simulink subsystem "PvtSubSys_VSM_LCKIE"  (R2020b)
settings: Solver=VariableStepAuto  StartTime=0.0  StopTime=10.0  RelTol=1e-3
values from neighbouring files (symbols this model uses):
  P_VSM_LCKIE_ClassInput = 0.0    [LCKIE.sldd]
  P_VSM_LCKIE_Laneoffset : value not decoded    [LCKIE.sldd]
  P_VSM_LCKIE_Laneoffset_BP : value not decoded    [LCKIE.sldd]
  P_VSM_LCKIE_LatC_DisOffofLanWidth : value not decoded    [LCKIE.sldd]
  P_VSM_LCKIE_LatC_DisOffofSpd : value not decoded    [LCKIE.sldd]
  P_VSM_LCKIE_LatC_DisSW = 0.0    [LCKIE.sldd]
  P_VSM_LCKIE_LatC_LanWidth : value not decoded    [LCKIE.sldd]
  P_VSM_LCKIE_LATC_LimitDis : value not decoded    [LCKIE.sldd]
  P_VSM_LCKIE_LATC_LimitDis_BP : value not decoded    [LCKIE.sldd]
  P_VSM_LCKIE_LatC_LimitDisEgoToObjSelt = 1.5    [LCKIE.sldd]
  P_VSM_LCKIE_LatC_LimitEgoToOppLane = 0.3    [LCKIE.sldd]
  P_VSM_LCKIE_LatC_maxLimitDisREToLane = 2.5    [LCKIE.sldd]
  P_VSM_LCKIE_LatC_minLimitDisREToLane = 1.2    [LCKIE.sldd]
  P_VSM_LCKIE_LatC_MoveEnableDis = 0.0    [LCKIE.sldd]
  P_VSM_LCKIE_LatC_RESafDis = 0.8    [LCKIE.sldd]
  P_VSM_LCKIE_LatC_SafeDisofLanWidth : value not decoded    [LCKIE.sldd]
  P_VSM_LCKIE_LatC_Spd : value not decoded    [LCKIE.sldd]
  P_VSM_LCKIE_LongC_d1 : value not decoded    [LCKIE.sldd]
  P_VSM_LCKIE_LongC_d2 : value not decoded    [LCKIE.sldd]
  P_VSM_LCKIE_LongC_DetaSpd : value not decoded    [LCKIE.sldd]
  P_VSM_LCKIE_LongC_DirecChangeDis = 20.0    [LCKIE.sldd]
  P_VSM_LCKIE_LongC_FleetOff = 80.0    [LCKIE.sldd]
  P_VSM_LCKIE_LongC_maxDis = 80.0    [LCKIE.sldd]
  P_VSM_LCKIE_LongC_minDis = 50.0    [LCKIE.sldd]
  P_VSM_LCKIE_LongC_ShutDownLongDis = -25.0    [LCKIE.sldd]
  P_VSM_LCKIE_LongC_ShutDownTTC = -4.0    [LCKIE.sldd]
  P_VSM_LCKIE_LongC_Spd : value not decoded    [LCKIE.sldd]
  P_VSM_LCKIE_LongC_toff = 10.0    [LCKIE.sldd]
  P_VSM_LCKIE_OFC_ActDis = 10.0    [LCKIE.sldd]
  P_VSM_LCKIE_OFC_DownDis = 10.0    [LCKIE.sldd]
  P_VSM_LCKIE_OFC_DownTTC = 5.0    [LCKIE.sldd]
  P_VSM_LCKIE_OFC_SafDis = 10.0    [LCKIE.sldd]
  P_VSM_LCKIE_OFC_Toff = 3.0    [LCKIE.sldd]
  P_VSM_LCKIE_ORC_LatDis = 1.8    [LCKIE.sldd]
  P_VSM_LCKIE_ORC_LimitDis1 = -30.0    [LCKIE.sldd]
  P_VSM_LCKIE_ORC_LimitDis2 = -10.0    [LCKIE.sldd]
  P_VSM_LCKIE_ORC_LimitTTC = 10.0    [LCKIE.sldd]
  P_VSM_LCKIE_ORC_LowSpd = -5.0    [LCKIE.sldd]
  P_VSM_LCKIE_POC_Delaytime : value not decoded    [LCKIE.sldd]
  P_VSM_LCKIE_POC_detaSpd : value not decoded    [LCKIE.sldd]
  P_VSM_LCKIE_POC_LimitDis = -15.0    [LCKIE.sldd]
  P_VSM_LCKIE_POC_LimitTTC = 2.0    [LCKIE.sldd]
  P_VSM_LCKIE_State_CurveMax = 0.005    [LCKIE.sldd]
  P_VSM_LCKIE_State_CurveMin = 0.0055555555555555558    [LCKIE.sldd]
  P_VSM_LCKIE_State_detaspd = 1.39    [LCKIE.sldd]
  P_VSM_LCKIE_State_detaspd_enable = 1.0    [LCKIE.sldd]
  P_VSM_LCKIE_State_DriverInputTrqValue_enable = 1.0    [LCKIE.sldd]
  P_VSM_LCKIE_State_ELKObjClc = 1.0    [LCKIE.sldd]
  P_VSM_LCKIE_State_HWASts_disable = 1.0    [LCKIE.sldd]
  P_VSM_LCKIE_State_IEObjClc = 1.0    [LCKIE.sldd]
  P_VSM_LCKIE_State_IFVReady = 1.0    [LCKIE.sldd]
  P_VSM_LCKIE_State_lamb_enable = 1.0    [LCKIE.sldd]
  P_VSM_LCKIE_State_Lanecurve_enable = 1.0    [LCKIE.sldd]
  P_VSM_LCKIE_State_LaneWidth_enable = 1.0    [LCKIE.sldd]
  P_VSM_LCKIE_State_Off2on = 3.0    [LCKIE.sldd]
  P_VSM_LCKIE_State_OppObjClc = 1.0    [LCKIE.sldd]
  P_VSM_LCKIE_STATE_ORCObjenable = 0.0    [LCKIE.sldd]
  P_VSM_LCKIE_State_Vehspeed_enable = 1.0    [LCKIE.sldd]
  P_VSM_LCKIE_State_wiper_enable = 1.0    [LCKIE.sldd]
  P_VSM_LCKIE_tcycle = 0.02    [LCKIE.sldd]
undefined symbols (not defined in the file or in its folder): P_Global_Vehicle_Length_m, P_Global_VehicleWidthMin_m, P_VSM_LSMC_SampleTime, STATE
libraries: simulink x62
(part 3 of 5)

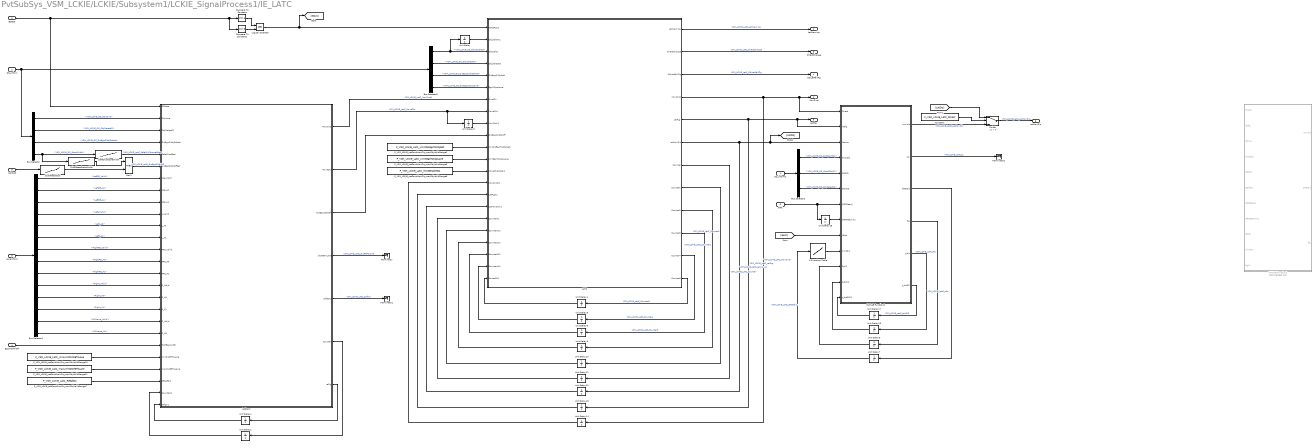
== system PvtSubSys_VSM_LCKIE/LCKIE/Subsystem1/LCKIE_SignalProcess1/IE_LATC ==
  OS_Inform : Inport
  IEstate : Inport  Port=2
  VehSpd : Inport  Port=3
  EgoHalfWidth : Inport  Port=4
  LaneInform : Inport  Port=5
  ORC : Inport  Port=6
  1-D Lookup Table : Lookup_n-D  NumberOfTableDimensions=1  BreakpointsForDimension1=P_VSM_LCKIE_LATC_LimitDis_BP  Table=P_VSM_LCKIE_LATC_LimitDis  InternalRulePriority=Speed  RndMeth=Simplest  InputSameDT=on
  Bus Selector : BusSelector  OutputSignals=VSM_LCKIE_OS_ObjLane,VSM_LCKIE_OS_ObjSelectID,VSM_LCKIE_OS_DisEgo2ObjSelect,VSM_LCKIE_OS_RoadWidth
  Bus Selector1 : BusSelector  OutputSignals=Lanes.LeftRE_Valid,Lanes.LeftRE_A0,Lanes.LeftRE_A1,Lanes.Left_Valid,Lanes.Left_A0,Lanes.Left_A1,Lanes.RightRE_Valid,Lanes.RightRE_A0,Lanes.RightRE_A1,Lanes.Right_Valid,Lanes.Right_A0,Lanes.Right_A1,Center.LCKLane_Valid,Center.LCKLane_A0
  Bus Selector2 : BusSelector  OutputSignals=VSM_LCKIE_OS_DisEgo2Obj,VSM_LCKIE_OS_OppRObjID,VSM_LCKIE_OS_ObjSelectID
  Bus Selector3 : BusSelector  OutputSignals=VSM_LCKIE_OS_ObjIDSelect,VSM_LCKIE_OS_ObjSelectID,VSM_LCKIE_OS_DisEgo2ObjSelect,VSM_LCKIE_OS_DisEgo2OppLane
  Compare To Constant : simulink/Logic and Bit Operations/Compare To Constant  relop===  const=4  OutDataTypeStr=boolean
  Compare To Constant1 : simulink/Logic and Bit Operations/Compare To Constant  relop===  const=5  OutDataTypeStr=boolean
  Constant : Constant  Value=P_VSM_LCKIE_LatC_DisSW
  DisOffsetofLaneWidth : Lookup_n-D  NumberOfTableDimensions=1  BreakpointsForDimension1=P_VSM_LCKIE_LatC_LanWidth  Table=P_VSM_LCKIE_LatC_DisOffofLanWidth  ExtrapMethod=Clip  UseLastTableValue=on  InternalRulePriority=Speed  RndMeth=Simplest  InputSameDT=on
  DisOffsetofSpd : Lookup_n-D  NumberOfTableDimensions=1  BreakpointsForDimension1=P_VSM_LCKIE_LatC_Spd  Table=P_VSM_LCKIE_LatC_DisOffofSpd  ExtrapMethod=Clip  UseLastTableValue=on  InternalRulePriority=Speed  RndMeth=Simplest  InputSameDT=on
  LATC : MATLAB Function  TreatAsAtomicUnit=on
  LatParm : MATLAB Function  TreatAsAtomicUnit=on
  Logical Operator : Logic  Operator=OR  AllPortsSameDT=off  OutDataTypeStr=boolean
  MATLAB Function1 : MATLAB Function  Commented=on  TreatAsAtomicUnit=on
  MATLAB Function2 : MATLAB Function  TreatAsAtomicUnit=on
  Max1 : MinMax  Function=max  Inputs=2
  OS_Inform1 : InportShadow
  P_VSM_LCKIE_LatConditionClc_maxObjValidRange10 : Constant  Value=P_VSM_LCKIE_LatC_minLimitDisREToLane
  P_VSM_LCKIE_LatConditionClc_maxObjValidRange11 : Constant  Value=P_VSM_LCKIE_LatC_maxLimitDisREToLane
  P_VSM_LCKIE_LatConditionClc_maxObjValidRange2 : Constant  Value=P_VSM_LCKIE_LatC_LimitDisEgoToObjSelt
  P_VSM_LCKIE_LatConditionClc_maxObjValidRange3 : Constant  Value=P_VSM_LCKIE_LatC_LimitEgoToOppLane
  P_VSM_LCKIE_LatConditionClc_maxObjValidRange7 : Constant  Value=P_VSM_LCKIE_LatC_RESafDis
  P_VSM_LCKIE_LatConditionClc_maxObjValidRange8 : Constant  Value=P_VSM_LCKIE_LatC_MoveEnableDis  OutDataTypeStr=single
  SafeDisofLaneWidth : Lookup_n-D  NumberOfTableDimensions=1  BreakpointsForDimension1=P_VSM_LCKIE_LatC_LanWidth  Table=P_VSM_LCKIE_LatC_SafeDisofLanWidth  ExtrapMethod=Clip  UseLastTableValue=on  InternalRulePriority=Speed  RndMeth=Simplest  InputSameDT=on
  Switch : Switch  Criteria=u2 > Threshold
  Terminator : Terminator
  Terminator1 : Terminator
  Terminator2 : Terminator
  Unit Delay{,1..17} (18 alike) : UnitDelay  SampleTime=-1  HasFrameUpgradeWarning=on
  MovDirct : Outport
  LatWarning : Outport  Port=2
  DirectChange : Outport  Port=3
  ObjLatFailFlg : Outport  Port=4
  LatFLg : Outport  Port=5
  LatMovDis : Outport  Port=6
  wires:
  DisOffsetofLaneWidth/1 -> Max1/1
  IEstate/1 -> LatParm/1(IEState), Compare To Constant1/1, Compare To Constant/1
  EgoHalfWidth/1 -> LatParm/21(HalfEgoWidth)
  Max1/1 -> LatParm/6(DisEgo2ObjOffset)  "VSM_LCKIE_LatC_DisEgo2ObjOff"
  SafeDisofLaneWidth/1 -> LatParm/5(SafeDisoffset)  "VSM_LCKIE_LatC_SafeDisToLaneEdge"
  Bus Selector/4 -> SafeDisofLaneWidth/1, DisOffsetofLaneWidth/1  "<VSM_LCKIE_OS_RoadWidth>"
  DisOffsetofSpd/1 -> Max1/2
  VehSpd/1 -> DisOffsetofSpd/1
  OS_Inform/1 -> Bus Selector3/1, Bus Selector/1
  Bus Selector/1 -> LatParm/2(ObjLane)  "<VSM_LCKIE_OS_ObjLane>"
  Bus Selector/2 -> LatParm/3(ObjSelectID)  "<VSM_LCKIE_OS_ObjSelectID>"
  LaneInform/1 -> Bus Selector1/1
  Bus Selector1/2 -> LatParm/8(LRe_A0)  "<LeftRE_A0>"
  Bus Selector1/3 -> LatParm/9(LRe_A1)  "<LeftRE_A1>"
  Bus Selector1/1 -> LatParm/7(LRe_Valid)  "<LeftRE_Valid>"
  Bus Selector1/4 -> LatParm/10(L_Valid)  "<Left_Valid>"
  Bus Selector1/5 -> LatParm/11(L_A0)  "<Left_A0>"
  Bus Selector1/6 -> LatParm/12(L_A1)  "<Left_A1>"
  Bus Selector1/7 -> LatParm/13(RRe_Valid)  "<RightRE_Valid>"
  Bus Selector1/8 -> LatParm/14(RRe_A0)  "<RightRE_A0>"
  Bus Selector1/9 -> LatParm/15(RRe_A1)  "<RightRE_A1>"
  Bus Selector1/10 -> LatParm/16(R_Valid)  "<Right_Valid>"
  Bus Selector1/11 -> LatParm/17(R_A0)  "<Right_A0>"
  Bus Selector1/12 -> LatParm/18(R_A1)  "<Right_A1>"
  Bus Selector1/13 -> LatParm/19(C_Valid)  "<LCKLane_Valid>"
  Bus Selector1/14 -> LatParm/20(C_A0)  "<LCKLane_A0>"
  P_VSM_LCKIE_LatConditionClc_maxObjValidRange10/1 -> LatParm/22(minDisREToLane)
  P_VSM_LCKIE_LatConditionClc_maxObjValidRange11/1 -> LatParm/23(maxDisREToLane)
  LatParm/7(reflg) -> Unit Delay1/1
  Unit Delay1/1 -> LatParm/26(reflgK1)
  Unit Delay2/1 -> LatParm/25(CounterK1)
  LatParm/6(Counter) -> Unit Delay2/1
  Bus Selector/3 -> LatParm/4(DisEgo2ObjSelect)  "<VSM_LCKIE_OS_DisEgo2ObjSelect>"
  P_VSM_LCKIE_LatConditionClc_maxObjValidRange7/1 -> LatParm/24(RESafDis)
  Bus Selector3/1 -> Unit Delay/1, LATC/3(ObjSelID)  "<VSM_LCKIE_OS_ObjIDSelect>"
  Bus Selector3/2 -> LATC/4(ObjSelectID)  "<VSM_LCKIE_OS_ObjSelectID>"
  Bus Selector3/3 -> LATC/5(DisEgo2ObjSelt)  "<VSM_LCKIE_OS_DisEgo2ObjSelect>"
  Bus Selector3/4 -> LATC/6(Ego2OppLane)  "<VSM_LCKIE_OS_DisEgo2OppLane>"
  Unit Delay/1 -> LATC/2(ObjSelIDK1)
  LatParm/1(MovDirct) -> LATC/7(DirctClc)  "VSM_LCKIE_LatC_MovDirct1"
  LatParm/2(MoveDis) -> Unit Delay3/1, LATC/8(MoveDis)  "VSM_LCKIE_LatC_MoveDis"
  LatParm/3(DisEgo2ObjOff) -> LATC/10(DisEgo2oObjOff)
  P_VSM_LCKIE_LatConditionClc_maxObjValidRange2/1 -> LATC/11(minDisEgoToObjSelt)
  P_VSM_LCKIE_LatConditionClc_maxObjValidRange3/1 -> LATC/12(minEgoToOppLane)
  P_VSM_LCKIE_LatConditionClc_maxObjValidRange8/1 -> LATC/13(MoveEnableDis)
  Unit Delay3/1 -> LATC/9(MovDisK1)
  LATC/12(Counter5) -> Unit Delay4/1  "VSM_LCKIE_LatC_Counter5"
  Unit Delay4/1 -> LATC/22(Couter5K1)
  LATC/11(Counter4) -> Unit Delay5/1  "VSM_LCKIE_LatC_Counter4"
  Unit Delay5/1 -> LATC/21(Counter4K1)
  LATC/10(Counter3) -> Unit Delay8/1  "VSM_LCKIE_LatC_Counter3"
  Unit Delay8/1 -> LATC/20(Counter3K1)
  LATC/9(Counter2) -> Unit Delay9/1  "VSM_LCKIE_LatC_Counter2"
  Unit Delay9/1 -> LATC/19(Counter2K1)
  LATC/8(Counter1) -> Unit Delay10/1  "VSM_LCKIE_LatC_Counter1"
  Unit Delay10/1 -> LATC/18(Counter1K1)
  LATC/7(Counter) -> Unit Delay11/1  "VSM_LCKIE_LatC_Counter"
  Unit Delay11/1 -> LATC/17(CounterK1)
  LATC/6(LatMovDis) -> Unit Delay12/1, MATLAB Function2/3(latmov), [LatDis]  "VSM_LCKIE_LatC_latmovori"
  Unit Delay12/1 -> LATC/16(LatMovDisK1)
  LATC/5(LatFLg) -> MATLAB Function2/2(latflg), LatFLg/1, Unit Delay13/1  "VSM_LCKIE_LatC_LatFLg"
  Unit Delay13/1 -> LATC/15(LatFLgK1)
  LATC/4(MovDirct) -> MATLAB Function2/1(Direct), MovDirct/1, Unit Delay14/1  "VSM_LCKIE_LatC_MovDirct"
  Unit Delay14/1 -> LATC/14(MovDirctK1)
  LatParm/4(DisREToLane) -> Terminator/1  "VSM_LCKIE_LatC_DisREToLane"
  LatParm/5(SafeDis) -> Terminator1/1  "VSM_LCKIE_LatC_SafDis"
  LATC/1(LatWarning) -> LatWarning/1  "VSM_LCKIE_LatC_LatWarning"
  LATC/2(DirectChange) -> DirectChange/1  "VSM_LCKIE_LatC_DirectChange"
  LATC/3(ObjLatFailFlg) -> ObjLatFailFlg/1  "VSM_LCKIE_LatC_ObjLatFailFlg"
  Compare To Constant/1 -> Logical Operator/1
  Compare To Constant1/1 -> Logical Operator/2
  Logical Operator/1 -> [IEAct], LATC/1(IEActFlgK1)
  MATLAB Function2/1(movdis) -> Switch/3  "VSM_LCKIE_LatC_LatMovDis"
  OS_Inform1/1 -> Bus Selector2/1
  Bus Selector2/2 -> MATLAB Function2/5(ORCID)  "<VSM_LCKIE_OS_OppRObjID>"
  Bus Selector2/1 -> MATLAB Function2/4(Dis2Obj)  "<VSM_LCKIE_OS_DisEgo2Obj>"
  Bus Selector2/3 -> MATLAB Function2/6(SelctID)  "<VSM_LCKIE_OS_ObjSelectID>"
  ORC/1 -> MATLAB Function2/7(ORCReady), Unit Delay15/1
  1-D Lookup Table/1 -> MATLAB Function2/10(limitDis)
  MATLAB Function2/4(flg) -> Unit Delay6/1  "VSM_LCKIE_LatC_Flg"
  Unit Delay6/1 -> MATLAB Function2/11(flgK1)
  MATLAB Function2/3(detaDis) -> Unit Delay7/1
  Unit Delay7/1 -> 1-D Lookup Table/1  "VSM_LCKIE_LatC_DetaDis"
  Unit Delay15/1 -> MATLAB Function2/8(ORCReadyK1)
  [IEAct] -> MATLAB Function2/9(IEAct)
  Constant/1 -> Switch/2
  Switch/1 -> LatMovDis/1  "VSM_LCKIE_LatC_LatMovDis"
  [LatDis] -> Switch/1
  MATLAB Function2/6(t_disOR) -> Unit Delay17/1  "VSM_LCKIE_LatC_tdisOR"
  Unit Delay17/1 -> MATLAB Function2/13(t_disORK1)
  MATLAB Function2/5(t_dis) -> Unit Delay16/1  "VSM_LCKIE_LatC_tdis"
  Unit Delay16/1 -> MATLAB Function2/12(t_disK1)
  MATLAB Function2/2(t_s) -> Terminator2/1  "VSM_LCKIE_LatC_ts"

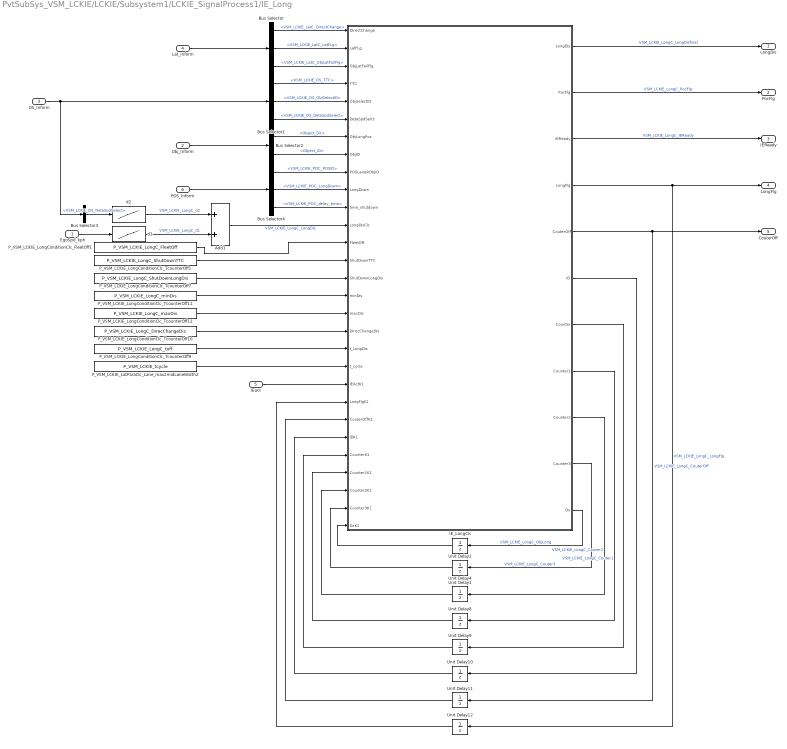
== system PvtSubSys_VSM_LCKIE/LCKIE/Subsystem1/LCKIE_SignalProcess1/IE_Long ==
  EgoSpd_kph : Inport
  Obj_Inform : Inport  Port=2
  OS_Inform : Inport  Port=3
  Lat_Inform : Inport  Port=4
  IEact : Inport  Port=5
  POS_Inform : Inport  Port=6
  Add1 : Sum
  Bus Selector : BusSelector  OutputSignals=VSM_LCKIE_LatC_DirectChange,VSM_LCKIE_LatC_LatFLg,VSM_LCKIE_LatC_ObjLatFailFlg
  Bus Selector1 : BusSelector  OutputSignals=VSM_LCKIE_OS_TTC,VSM_LCKIE_OS_ObjSelectID,VSM_LCKIE_OS_DetaSpdSelect
  Bus Selector2 : BusSelector  OutputSignals=Object_DX,Object_ID
  Bus Selector3 : BusSelector  OutputSignals=VSM_LCKIE_OS_DetaSpdSelect
  Bus Selector4 : BusSelector  OutputSignals=VSM_LCKIE_POC_POSID,VSM_LCKIE_POC_LongDown,VSM_LCKIE_POC_delay_time
  IE_LongClc : MATLAB Function  TreatAsAtomicUnit=on
  P_VSM_LCKIE_LatParaClc_Lane_max2midLaneWidth2 : Constant  Value=P_VSM_LCKIE_tcycle
  P_VSM_LCKIE_LongConditionClc_FleetOff1 : Constant  Value=P_VSM_LCKIE_LongC_FleetOff
  P_VSM_LCKIE_LongConditionClc_TcounterOff1 : Constant  Value=P_VSM_LCKIE_LongC_ShutDownTTC
  P_VSM_LCKIE_LongConditionClc_TcounterOff10 : Constant  Value=P_VSM_LCKIE_LongC_DirecChangeDis
  P_VSM_LCKIE_LongConditionClc_TcounterOff11 : Constant  Value=P_VSM_LCKIE_LongC_minDis
  P_VSM_LCKIE_LongConditionClc_TcounterOff12 : Constant  Value=P_VSM_LCKIE_LongC_maxDis
  P_VSM_LCKIE_LongConditionClc_TcounterOff7 : Constant  Value=P_VSM_LCKIE_LongC_ShutDownLongDis
  P_VSM_LCKIE_LongConditionClc_TcounterOff9 : Constant  Value=P_VSM_LCKIE_LongC_toff
  Unit Delay{1..2,4,8..12} (8 alike) : UnitDelay  SampleTime=-1  HasFrameUpgradeWarning=on
  d1 : Lookup_n-D  NumberOfTableDimensions=1  BreakpointsForDimension1=P_VSM_LCKIE_LongC_Spd  Table=P_VSM_LCKIE_LongC_d1  ExtrapMethod=Clip  UseLastTableValue=on  InternalRulePriority=Speed  RndMeth=Simplest  InputSameDT=on
  d2 : Lookup_n-D  NumberOfTableDimensions=1  BreakpointsForDimension1=P_VSM_LCKIE_LongC_DetaSpd  Table=P_VSM_LCKIE_LongC_d2  ExtrapMethod=Clip  UseLastTableValue=on  InternalRulePriority=Speed  OutDataTypeStr=single  RndMeth=Simplest  InputSameDT=on
  LongDis : Outport
  PocFlg : Outport  Port=2
  IEReady : Outport  Port=3
  LongFlg : Outport  Port=4
  CouterOff : Outport  Port=5
  wires:
  Bus Selector3/1 -> d2/1  "<VSM_LCKIE_OS_DetaSpdSelect>"
  EgoSpd_kph/1 -> d1/1
  d2/1 -> Add1/1  "VSM_LCKIE_LongC_d2"
  d1/1 -> Add1/2  "VSM_LCKIE_LongC_d1"
  Add1/1 -> IE_LongClc/12(LongDisClc)  "VSM_LCKIE_LongC_LongDis"
  Lat_Inform/1 -> Bus Selector/1
  OS_Inform/1 -> Bus Selector1/1, Bus Selector3/1
  P_VSM_LCKIE_LongConditionClc_TcounterOff1/1 -> IE_LongClc/14(ShutDownTTC)
  P_VSM_LCKIE_LongConditionClc_TcounterOff7/1 -> IE_LongClc/15(ShutDownLongDis)
  P_VSM_LCKIE_LongConditionClc_TcounterOff9/1 -> IE_LongClc/19(t_LongDis)
  P_VSM_LCKIE_LatParaClc_Lane_max2midLaneWidth2/1 -> IE_LongClc/20(t_cycle)
  IE_LongClc/10(Counter3) -> Unit Delay4/1  "VSM_LCKIE_LongC_Couter3"
  Unit Delay4/1 -> IE_LongClc/28(Counter3K1)
  IE_LongClc/9(Counter2) -> Unit Delay1/1  "VSM_LCKIE_LongC_Couter2"
  Unit Delay1/1 -> IE_LongClc/27(Counter2K1)
  IE_LongClc/8(Counter1) -> Unit Delay8/1  "VSM_LCKIE_LongC_Couter1"
  Unit Delay8/1 -> IE_LongClc/26(Counter1K1)
  IE_LongClc/7(Counter) -> Unit Delay9/1
  Unit Delay9/1 -> IE_LongClc/25(CounterK1)
  IE_LongClc/6(ID) -> Unit Delay10/1
  Unit Delay10/1 -> IE_LongClc/24(IDK1)
  IE_LongClc/5(CouterOff) -> CouterOff/1, Unit Delay11/1  "VSM_LCKIE_LongC_CouterOff"
  Unit Delay11/1 -> IE_LongClc/23(CouterOffK1)
  IE_LongClc/4(LongFlg) -> LongFlg/1, Unit Delay12/1  "VSM_LCKIE_LongC_LongFlg"
  Unit Delay12/1 -> IE_LongClc/22(LongFlgK1)
  IE_LongClc/3(IEReady) -> IEReady/1  "VSM_LCKIE_LongC_IEReady"
  Bus Selector/2 -> IE_LongClc/2(LatFLg)  "<VSM_LCKIE_LatC_LatFLg>"
  Bus Selector/3 -> IE_LongClc/3(ObjLatFailFlg)  "<VSM_LCKIE_LatC_ObjLatFailFlg>"
  Bus Selector1/2 -> IE_LongClc/5(ObjSelectID)  "<VSM_LCKIE_OS_ObjSelectID>"
  Bus Selector1/3 -> IE_LongClc/6(DetaSpdSelct)  "<VSM_LCKIE_OS_DetaSpdSelect>"
  Bus Selector1/1 -> IE_LongClc/4(TTC)  "<VSM_LCKIE_OS_TTC>"
  Obj_Inform/1 -> Bus Selector2/1
  Bus Selector2/2 -> IE_LongClc/8(ObjID)  "<Object_ID>"
  Bus Selector2/1 -> IE_LongClc/7(ObjLongPos)  "<Object_DX>"
  POS_Inform/1 -> Bus Selector4/1
  IE_LongClc/1(LongDis) -> LongDis/1  "VSM_LCKIE_LongC_LongDisfinal"
  IE_LongClc/2(PocFlg) -> PocFlg/1  "VSM_LCKIE_LongC_PocFlg"
  IE_LongClc/11(Dx) -> Unit Delay2/1  "VSM_LCKIE_LongC_ObjLong"
  P_VSM_LCKIE_LongConditionClc_FleetOff1/1 -> IE_LongClc/13(FleetOff)
  Unit Delay2/1 -> IE_LongClc/29(DxK1)
  P_VSM_LCKIE_LongConditionClc_TcounterOff11/1 -> IE_LongClc/16(minDis)
  P_VSM_LCKIE_LongConditionClc_TcounterOff12/1 -> IE_LongClc/17(maxDis)
  P_VSM_LCKIE_LongConditionClc_TcounterOff10/1 -> IE_LongClc/18(DirecChangeDis)
  Bus Selector4/1 -> IE_LongClc/9(POSLaneRObjID)  "<VSM_LCKIE_POC_POSID>"
  Bus Selector4/2 -> IE_LongClc/10(LongDown)  "<VSM_LCKIE_POC_LongDown>"
  Bus Selector4/3 -> IE_LongClc/11(time_shutdown)  "<VSM_LCKIE_POC_delay_time>"
  Bus Selector/1 -> IE_LongClc/1(DirectChange)  "<VSM_LCKIE_LatC_DirectChange>"
  IEact/1 -> IE_LongClc/21(IEActK1)

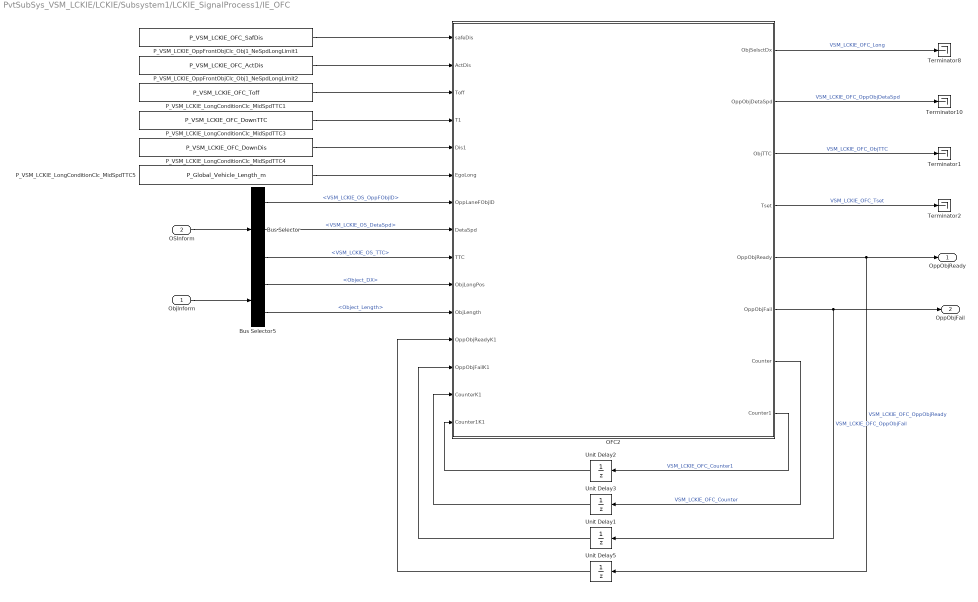
== system PvtSubSys_VSM_LCKIE/LCKIE/Subsystem1/LCKIE_SignalProcess1/IE_OFC ==
  ObjInform : Inport
  OSInform : Inport  Port=2
  Bus Selector : BusSelector  OutputSignals=VSM_LCKIE_OS_OppFObjID,VSM_LCKIE_OS_DetaSpd,VSM_LCKIE_OS_TTC
  Bus Selector5 : BusSelector  OutputSignals=Object_DX,Object_Length
  OFC2 : MATLAB Function  TreatAsAtomicUnit=on
  P_VSM_LCKIE_LongConditionClc_MidSpdTTC1 : Constant  Value=P_VSM_LCKIE_OFC_Toff
  P_VSM_LCKIE_LongConditionClc_MidSpdTTC3 : Constant  Value=P_VSM_LCKIE_OFC_DownTTC
  P_VSM_LCKIE_LongConditionClc_MidSpdTTC4 : Constant  Value=P_VSM_LCKIE_OFC_DownDis
  P_VSM_LCKIE_LongConditionClc_MidSpdTTC5 : Constant  Value=P_Global_Vehicle_Length_m
  P_VSM_LCKIE_OppFrontObjClc_Obj1_NeSpdLongLimit1 : Constant  Value=P_VSM_LCKIE_OFC_SafDis
  P_VSM_LCKIE_OppFrontObjClc_Obj1_NeSpdLongLimit2 : Constant  Value=P_VSM_LCKIE_OFC_ActDis
  Terminator{1..2,8,10} (4 alike) : Terminator
  Unit Delay{1..3,5} (4 alike) : UnitDelay  SampleTime=-1  HasFrameUpgradeWarning=on
  OppObjReady : Outport
  OppObjFail : Outport  Port=2
  wires:
  OFC2/3(ObjTTC) -> Terminator1/1  "VSM_LCKIE_OFC_ObjTTC"
  Unit Delay2/1 -> OFC2/15(Counter1K1)
  OFC2/8(Counter1) -> Unit Delay2/1  "VSM_LCKIE_OFC_Counter1"
  Bus Selector/3 -> OFC2/9(TTC)  "<VSM_LCKIE_OS_TTC>"
  Bus Selector/2 -> OFC2/8(DetaSpd)  "<VSM_LCKIE_OS_DetaSpd>"
  Bus Selector/1 -> OFC2/7(OppLaneFObjID)  "<VSM_LCKIE_OS_OppFObjID>"
  OSInform/1 -> Bus Selector/1
  Unit Delay5/1 -> OFC2/12(OppObjReadyK1)
  Unit Delay1/1 -> OFC2/13(OppObjFailK1)
  OFC2/2(OppObjDetaSpd) -> Terminator10/1  "VSM_LCKIE_OFC_OppObjDetaSpd"
  OFC2/6(OppObjFail) -> Unit Delay1/1, OppObjFail/1  "VSM_LCKIE_OFC_OppObjFail"
  OFC2/4(Tset) -> Terminator2/1  "VSM_LCKIE_OFC_Tset"
  Bus Selector5/1 -> OFC2/10(ObjLongPos)  "<Object_DX>"
  OFC2/1(ObjSelsctDx) -> Terminator8/1  "VSM_LCKIE_OFC_Long"
  Bus Selector5/2 -> OFC2/11(ObjLength)  "<Object_Length>"
  Unit Delay3/1 -> OFC2/14(CounterK1)
  ObjInform/1 -> Bus Selector5/1
  P_VSM_LCKIE_OppFrontObjClc_Obj1_NeSpdLongLimit1/1 -> OFC2/1(safeDis)
  P_VSM_LCKIE_LongConditionClc_MidSpdTTC4/1 -> OFC2/5(Dis1)
  OFC2/7(Counter) -> Unit Delay3/1  "VSM_LCKIE_OFC_Counter"
  P_VSM_LCKIE_LongConditionClc_MidSpdTTC3/1 -> OFC2/4(T1)
  P_VSM_LCKIE_OppFrontObjClc_Obj1_NeSpdLongLimit2/1 -> OFC2/2(ActDis)
  P_VSM_LCKIE_LongConditionClc_MidSpdTTC5/1 -> OFC2/6(EgoLong)
  P_VSM_LCKIE_LongConditionClc_MidSpdTTC1/1 -> OFC2/3(Toff)
  OFC2/5(OppObjReady) -> Unit Delay5/1, OppObjReady/1  "VSM_LCKIE_OFC_OppObjReady"

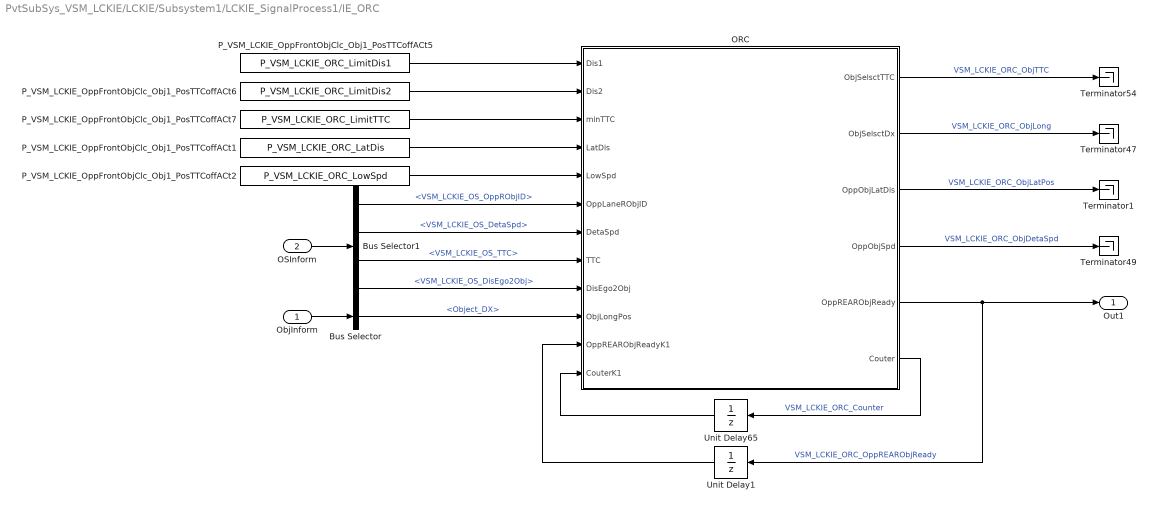
== system PvtSubSys_VSM_LCKIE/LCKIE/Subsystem1/LCKIE_SignalProcess1/IE_ORC ==
  ObjInform : Inport
  OSInform : Inport  Port=2
  Bus Selector : BusSelector  OutputSignals=Object_DX
  Bus Selector1 : BusSelector  OutputSignals=VSM_LCKIE_OS_OppRObjID,VSM_LCKIE_OS_DetaSpd,VSM_LCKIE_OS_TTC,VSM_LCKIE_OS_DisEgo2Obj
  ORC : MATLAB Function  TreatAsAtomicUnit=on
  P_VSM_LCKIE_OppFrontObjClc_Obj1_PosTTCoffACt1 : Constant  Value=P_VSM_LCKIE_ORC_LatDis
  P_VSM_LCKIE_OppFrontObjClc_Obj1_PosTTCoffACt2 : Constant  Value=P_VSM_LCKIE_ORC_LowSpd
  P_VSM_LCKIE_OppFrontObjClc_Obj1_PosTTCoffACt5 : Constant  Value=P_VSM_LCKIE_ORC_LimitDis1
  P_VSM_LCKIE_OppFrontObjClc_Obj1_PosTTCoffACt6 : Constant  Value=P_VSM_LCKIE_ORC_LimitDis2
  P_VSM_LCKIE_OppFrontObjClc_Obj1_PosTTCoffACt7 : Constant  Value=P_VSM_LCKIE_ORC_LimitTTC
  Terminator{1,47,49,54} (4 alike) : Terminator
  Unit Delay1 : UnitDelay  SampleTime=-1  HasFrameUpgradeWarning=on
  Unit Delay65 : UnitDelay  SampleTime=-1  HasFrameUpgradeWarning=on
  Out1 : Outport
  wires:
  Unit Delay1/1 -> ORC/11(OppREARObjReadyK1)
  Unit Delay65/1 -> ORC/12(CouterK1)
  Bus Selector1/3 -> ORC/8(TTC)  "<VSM_LCKIE_OS_TTC>"
  Bus Selector1/1 -> ORC/6(OppLaneRObjID)  "<VSM_LCKIE_OS_OppRObjID>"
  Bus Selector1/2 -> ORC/7(DetaSpd)  "<VSM_LCKIE_OS_DetaSpd>"
  OSInform/1 -> Bus Selector1/1
  Bus Selector/1 -> ORC/10(ObjLongPos)  "<Object_DX>"
  ObjInform/1 -> Bus Selector/1
  ORC/4(OppObjSpd) -> Terminator49/1  "VSM_LCKIE_ORC_ObjDetaSpd"
  ORC/6(Couter) -> Unit Delay65/1  "VSM_LCKIE_ORC_Counter"
  P_VSM_LCKIE_OppFrontObjClc_Obj1_PosTTCoffACt6/1 -> ORC/2(Dis2)
  ORC/5(OppREARObjReady) -> Out1/1, Unit Delay1/1  "VSM_LCKIE_ORC_OppREARObjReady"
  P_VSM_LCKIE_OppFrontObjClc_Obj1_PosTTCoffACt7/1 -> ORC/3(minTTC)
  ORC/1(ObjSelsctTTC) -> Terminator54/1  "VSM_LCKIE_ORC_ObjTTC"
  ORC/2(ObjSelsctDx) -> Terminator47/1  "VSM_LCKIE_ORC_ObjLong"
  P_VSM_LCKIE_OppFrontObjClc_Obj1_PosTTCoffACt5/1 -> ORC/1(Dis1)
  Bus Selector1/4 -> ORC/9(DisEgo2Obj)  "<VSM_LCKIE_OS_DisEgo2Obj>"
  P_VSM_LCKIE_OppFrontObjClc_Obj1_PosTTCoffACt1/1 -> ORC/4(LatDis)
  P_VSM_LCKIE_OppFrontObjClc_Obj1_PosTTCoffACt2/1 -> ORC/5(LowSpd)
  ORC/3(OppObjLatDis) -> Terminator1/1  "VSM_LCKIE_ORC_ObjLatPos"

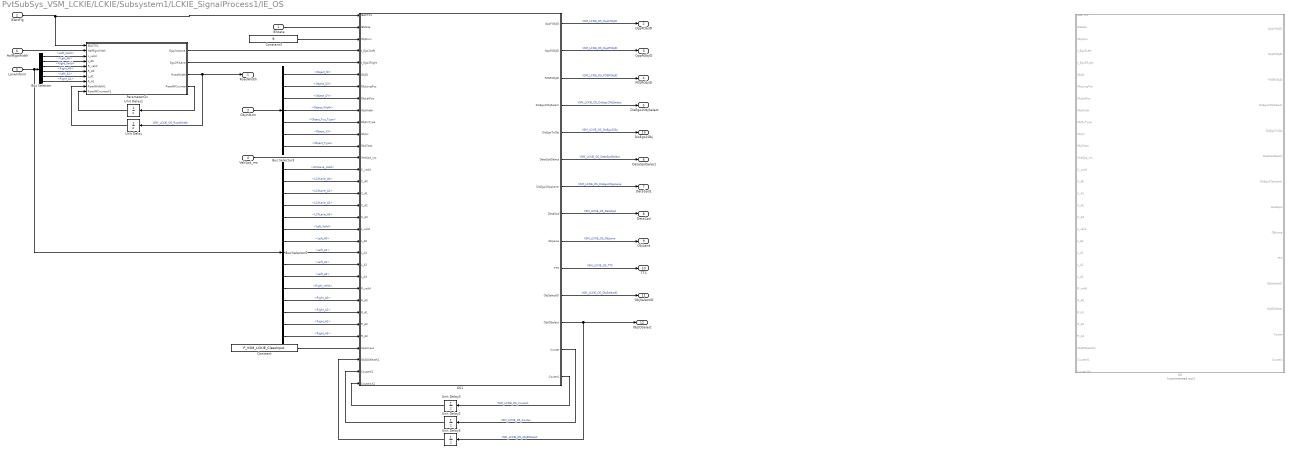
== system PvtSubSys_VSM_LCKIE/LCKIE/Subsystem1/LCKIE_SignalProcess1/IE_OS ==
  IEState : Inport
  IEActFlg : Inport  Port=2
  ObjInform : Inport  Port=3
  VehSpd_ms : Inport  Port=4
  LaneInform : Inport  Port=5
  HalfEgoWidth : Inport  Port=6
  Bus Selector : BusSelector  OutputSignals=Lanes.Left_Valid,Lanes.Left_A0,Lanes.Right_Valid,Lanes.Right_A0,Lanes.Left_A1,Lanes.Right_A1
  Bus Selector3 : BusSelector  OutputSignals=Object_ID,Object_DX,Object_DY,Object_Width,Object_Fus_Type,Object_VX,Object_Type
  Bus Selector5 : BusSelector  OutputSignals=Center.LCKLane_Valid,Center.LCKLane_A0,Center.LCKLane_A1,Center.LCKLane_A2,Center.LCKLane_A3,Lanes.Left_Valid,Lanes.Left_A0,Lanes.Left_A1,Lanes.Left_A2,Lanes.Left_A3,Lanes.Right_Valid,Lanes.Right_A0,Lanes.Right_A1,Lanes.Right_A2,Lanes.Right_A3
  Constant : Constant  Value=P_VSM_LCKIE_ClassInput
  Constant3 : Constant  Value=9  OutDataTypeStr=uint8
  OS : MATLAB Function  Commented=on  TreatAsAtomicUnit=on
  OS1 : MATLAB Function  TreatAsAtomicUnit=on
  ParameterClc : MATLAB Function  TreatAsAtomicUnit=on
  Unit Delay{,1..3,5} (5 alike) : UnitDelay  SampleTime=-1  HasFrameUpgradeWarning=on
  RoadWidth : Outport
  OppFObjID : Outport  Port=2
  OppRObjID : Outport  Port=3
  POSRObjID : Outport  Port=4
  DisEgo2ObjSelect : Outport  Port=5
  DetaSpdSelect : Outport  Port=6
  DetaSpd1 : Outport  Port=7
  DetaSpd : Outport  Port=8
  ObjLane : Outport  Port=9
  TTC : Outport  Port=10
  ObjSelectID : Outport  Port=11
  ObjIDSelect : Outport  Port=12
  DisEgo2Obj : Outport  Port=13
  wires:
  Unit Delay/1 -> ParameterClc/9(RoadWidthK1)
  Bus Selector3/3 -> OS1/8(ObjLatPos)  "<Object_DY>"
  ParameterClc/3(RoadWidth) -> RoadWidth/1, Unit Delay/1  "VSM_LCKIE_OS_RoadWidth"
  Unit Delay5/1 -> OS1/30(ObjIDSelectK1)
  Bus Selector/4 -> ParameterClc/6(R_A0)  "<Right_A0>"
  Unit Delay3/1 -> OS1/32(Couter1K1)
  ObjInform/1 -> Bus Selector3/1
  Bus Selector3/2 -> OS1/7(ObjLongPos)  "<Object_DX>"
  Unit Delay2/1 -> OS1/31(CouterK1)
  OS1/13(Couter) -> Unit Delay2/1  "VSM_LCKIE_OS_Couter"
  Bus Selector3/1 -> OS1/6(ObjID)  "<Object_ID>"
  Bus Selector/5 -> ParameterClc/7(L_A1)  "<Left_A1>"
  OS1/11(ObjSelectID) -> ObjSelectID/1  "VSM_LCKIE_OS_ObjSelectID"
  OS1/3(POSRObjID) -> POSRObjID/1  "VSM_LCKIE_OS_POSRObjID"
  HalfEgoWidth/1 -> ParameterClc/2(HalfEgoWidth)
  Bus Selector5/10 -> OS1/23(L_A3)  "<Left_A3>"
  Bus Selector/1 -> ParameterClc/3(L_valid)  "<Left_Valid>"
  OS1/2(OppRObjID) -> OppRObjID/1  "VSM_LCKIE_OS_OppRObjID"
  Bus Selector/3 -> ParameterClc/5(R_valid)  "<Right_Valid>"
  ParameterClc/1(Ego2LeLane) -> OS1/4(t_Ego2Left)
  Unit Delay1/1 -> ParameterClc/10(RoadWCounterK1)
  Bus Selector5/15 -> OS1/28(R_A3)  "<Right_A3>"
  Bus Selector5/12 -> OS1/25(R_A0)  "<Right_A0>"
  ParameterClc/4(RoadWCounter) -> Unit Delay1/1
  OS1/12(ObjIDSelect) -> Unit Delay5/1, ObjIDSelect/1  "VSM_LCKIE_OS_ObjIDSelect"
  Bus Selector/2 -> ParameterClc/4(L_A0)  "<Left_A0>"
  OS1/1(OppFObjID) -> OppFObjID/1  "VSM_LCKIE_OS_OppFObjID"
  LaneInform/1 -> Bus Selector5/1, Bus Selector/1
  Bus Selector/6 -> ParameterClc/8(R_A1)  "<Right_A1>"
  Bus Selector5/13 -> OS1/26(R_A1)  "<Right_A1>"
  Bus Selector3/7 -> OS1/12(ObjClass)  "<Object_Type>"
  OS1/14(Couter1) -> Unit Delay3/1  "VSM_LCKIE_OS_Couter1"
  Bus Selector3/4 -> OS1/9(ObjWidth)  "<Object_Width>"
  Bus Selector5/11 -> OS1/24(R_valid)  "<Right_Valid>"
  Bus Selector5/6 -> OS1/19(L_valid)  "<Left_Valid>"
  Bus Selector3/6 -> OS1/11(ObjVx)  "<Object_VX>"
  Bus Selector3/5 -> OS1/10(ObjFuType)  "<Object_Fus_Type>"
  Bus Selector5/9 -> OS1/22(L_A2)  "<Left_A2>"
  IEState/1 -> OS1/2(IEState)
  OS1/4(DisEgo2ObjSelect) -> DisEgo2ObjSelect/1  "VSM_LCKIE_OS_DisEgo2ObjSelect"
  VehSpd_ms/1 -> OS1/13(VheSpd_ms)
  OS1/10(TTC) -> TTC/1  "VSM_LCKIE_OS_TTC"
  ParameterClc/2(Ego2RiLane) -> OS1/5(t_Ego2Right)
  Bus Selector5/7 -> OS1/20(L_A0)  "<Left_A0>"
  OS1/6(DetaSpdSelect) -> DetaSpdSelect/1  "VSM_LCKIE_OS_DetaSpdSelect"
  Bus Selector5/8 -> OS1/21(L_A1)  "<Left_A1>"
  Bus Selector5/14 -> OS1/27(R_A2)  "<Right_A2>"
  Constant3/1 -> OS1/3(ObjNum)
  IEActFlg/1 -> OS1/1(IEACTK1), ParameterClc/1(IEACTK1)
  OS1/9(ObjLane) -> ObjLane/1  "VSM_LCKIE_OS_ObjLane"
  OS1/8(DetaSpd) -> DetaSpd/1  "VSM_LCKIE_OS_DetaSpd"
  Bus Selector5/1 -> OS1/14(C_valid)  "<LCKLane_Valid>"
  Bus Selector5/2 -> OS1/15(C_A0)  "<LCKLane_A0>"
  Bus Selector5/3 -> OS1/16(C_A1)  "<LCKLane_A1>"
  Bus Selector5/4 -> OS1/17(C_A2)  "<LCKLane_A2>"
  Bus Selector5/5 -> OS1/18(C_A3)  "<LCKLane_A3>"
  OS1/7(DisEgo2OppLane) -> DetaSpd1/1  "VSM_LCKIE_OS_DisEgo2OppLane"
  OS1/5(DisEgoToObj) -> DisEgo2Obj/1  "VSM_LCKIE_OS_DisEgo2Obj"
  Constant/1 -> OS1/29(classinput)

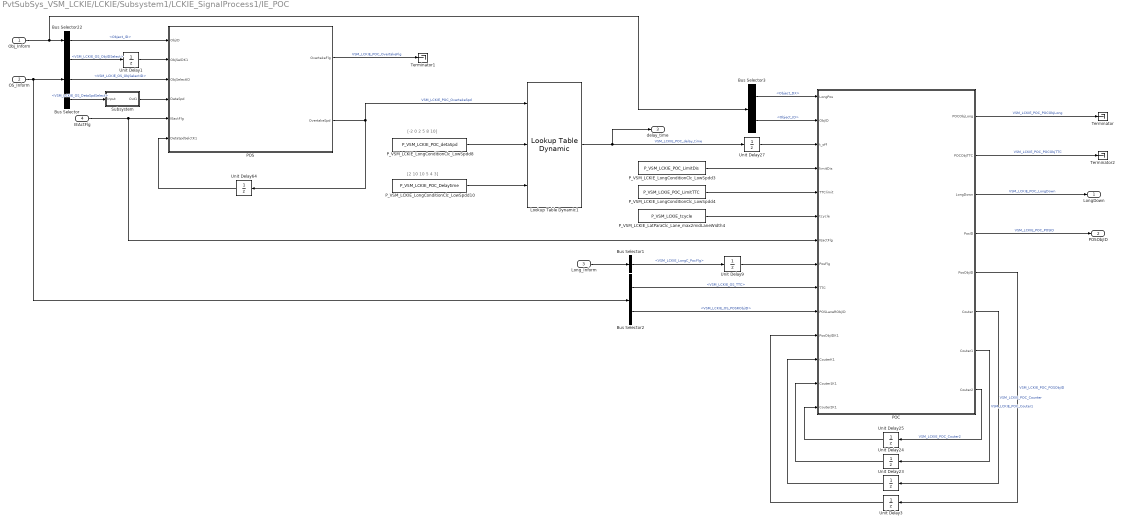
== system PvtSubSys_VSM_LCKIE/LCKIE/Subsystem1/LCKIE_SignalProcess1/IE_POC ==
  note: [2 10 10 5 4 3]
  note: [-2 0 2 5 8 10]
  Obj_Inform : Inport
  OS_Inform : Inport  Port=2
  Long_Inform : Inport  Port=3
  IEActFlg : Inport  Port=4
  Bus Selector : BusSelector  OutputSignals=VSM_LCKIE_OS_ObjIDSelect,VSM_LCKIE_OS_ObjSelectID,VSM_LCKIE_OS_DetaSpdSelect
  Bus Selector1 : BusSelector  OutputSignals=VSM_LCKIE_LongC_PocFlg
  Bus Selector2 : BusSelector  OutputSignals=VSM_LCKIE_OS_TTC,VSM_LCKIE_OS_POSRObjID
  Bus Selector22 : BusSelector  OutputSignals=Object_ID
  Bus Selector3 : BusSelector  OutputSignals=Object_DX,Object_ID
  Lookup Table Dynamic1 : simulink/Lookup Tables/Lookup Table Dynamic  LookUpMeth=Interpolation-Use End Values  OutDataType=fixdt('single')  OutScaling=[]  OutDataTypeStr=Inherit: Inherit via back propagation  DoSatur=off
  POC : MATLAB Function  TreatAsAtomicUnit=on
  POS : MATLAB Function  TreatAsAtomicUnit=on
  P_VSM_LCKIE_LatParaClc_Lane_max2midLaneWidth4 : Constant  Value=P_VSM_LCKIE_tcycle
  P_VSM_LCKIE_LongConditionClc_LowSpdd10 : Constant  Value=P_VSM_LCKIE_POC_Delaytime
  P_VSM_LCKIE_LongConditionClc_LowSpdd3 : Constant  Value=P_VSM_LCKIE_POC_LimitDis
  P_VSM_LCKIE_LongConditionClc_LowSpdd4 : Constant  Value=P_VSM_LCKIE_POC_LimitTTC
  P_VSM_LCKIE_LongConditionClc_LowSpdd8 : Constant  Value=P_VSM_LCKIE_POC_detaSpd  VectorParams1D=off
  Subsystem : Subsystem
  Terminator : Terminator
  Terminator1 : Terminator
  Terminator2 : Terminator
  Unit Delay{1,3,9,23..25,27,64} (8 alike) : UnitDelay  SampleTime=-1  HasFrameUpgradeWarning=on
  LongDown : Outport
  POSObjID : Outport  Port=2
  delay_time : Outport  Port=3
  wires:
  Bus Selector3/2 -> POC/2(ObjID)  "<Object_ID>"
  POC/5(PosObjID) -> Unit Delay3/1  "VSM_LCKIE_POC_POSObjID"
  POC/2(POCObjTTC) -> Terminator2/1  "VSM_LCKIE_POC_POCObjTTC"
  POC/1(POCObjLong) -> Terminator/1  "VSM_LCKIE_POC_POCObjLong"
  Bus Selector3/1 -> POC/1(LongPos)  "<Object_DX>"
  Bus Selector2/2 -> POC/10(POSLaneRObjID)  "<VSM_LCKIE_OS_POSRObjID>"
  Bus Selector2/1 -> POC/9(TTC)  "<VSM_LCKIE_OS_TTC>"
  OS_Inform/1 -> Bus Selector/1, Bus Selector2/1
  IEActFlg/1 -> POS/5(IEactFlg), POC/7(IEactFlg)
  Bus Selector1/1 -> Unit Delay9/1  "<VSM_LCKIE_LongC_PocFlg>"
  Long_Inform/1 -> Bus Selector1/1
  Unit Delay1/1 -> POS/2(ObjSeIDK1)
  Bus Selector/3 -> Subsystem/1(Input)  "<VSM_LCKIE_OS_DetaSpdSelect>"
  Bus Selector/2 -> POS/3(ObjSelectID)  "<VSM_LCKIE_OS_ObjSelectID>"
  Bus Selector/1 -> Unit Delay1/1  "<VSM_LCKIE_OS_ObjIDSelect>"
  Unit Delay25/1 -> POC/14(Couter2K1)
  P_VSM_LCKIE_LongConditionClc_LowSpdd3/1 -> POC/4(limitDis)
  Unit Delay23/1 -> POC/12(CouterK1)
  POS/1(OvertakeFlg) -> Terminator1/1  "VSM_LCKIE_POC_OvertakeFlg"
  Unit Delay64/1 -> POS/6(DetaSpdSelctK1)
  Obj_Inform/1 -> Bus Selector22/1, Bus Selector3/1
  Unit Delay24/1 -> POC/13(Couter1K1)
  POC/4(PosID) -> POSObjID/1  "VSM_LCKIE_POC_POSID"
  POC/8(Couter2) -> Unit Delay25/1  "VSM_LCKIE_POC_Couter2"
  Unit Delay9/1 -> POC/8(PosFlg)
  P_VSM_LCKIE_LatParaClc_Lane_max2midLaneWidth4/1 -> POC/6(tcycle)
  POC/3(LongDown) -> LongDown/1  "VSM_LCKIE_POC_LongDown"
  POC/7(Couter1) -> Unit Delay24/1  "VSM_LCKIE_POC_Couter1"
  P_VSM_LCKIE_LongConditionClc_LowSpdd10/1 -> Lookup Table Dynamic1/3
  P_VSM_LCKIE_LongConditionClc_LowSpdd4/1 -> POC/5(TTClimit)
  Lookup Table Dynamic1/1 -> Unit Delay27/1, delay_time/1  "VSM_LCKIE_POC_delay_time"
  POS/2(OvertakeSpd) -> Unit Delay64/1, Lookup Table Dynamic1/1  "VSM_LCKIE_POC_OvertakeSpd"
  P_VSM_LCKIE_LongConditionClc_LowSpdd8/1 -> Lookup Table Dynamic1/2
  Unit Delay3/1 -> POC/11(PosObjIDK1)
  Bus Selector22/1 -> POS/1(ObjID)  "<Object_ID>"
  Unit Delay27/1 -> POC/3(t_off)
  POC/6(Couter) -> Unit Delay23/1  "VSM_LCKIE_POC_Counter"
  Subsystem/1(Out1) -> POS/4(DetaSpd)
